simulink library "MotionBaseAdaptersLib"  (R2019b)
settings: Solver=VariableStepAuto  StartTime=0.0  StopTime=10.0  RelTol=1e-3
undefined symbols (not defined in the file): AngularAcceleration, AngularVelocity, ApplyMotion, DiscIntNeverNeededParam, GravitationalAcceleration, LinearAcceleration, LinearVelocity, ManualOrientation, ManualPosition, OrientationDCM, SampleTime, TrackEffectType
libraries: simulink x34, FiltersLib x34, OverridesLib x10, SignalGeneratorsLib x7, LatchesLib x6, TimersLib x5, CoordinateMathOperationsLib x2, MathOperationsLib x2, $bdroot x1
(part 2 of 2)

== system MotionBaseAdaptersLib/MotionBase/MotionBaseAdapter/MotionBaseProcessing/ManualAdjustments/ManualPositionAdjustment1/If Action Subsystem3 ==
  RoughnessProfileFactor : Inport
  Linear Velocity : Inport  Port=2
  RoughnessProfileFrequencyFactor : Inport  Port=3
  Action Port : ActionPort
  AssignZ : Assignment  IndexMode=Zero-based  DiagnosticForDimensions=Warning  IndexOptions=Index vector (dialog)  Indices=2  OutputSizes=1
  Compare To Zero : simulink/Logic and Bit Operations/Compare To Zero  relop=>  OutDataTypeStr=boolean
  Constant : Constant  Value=1/20
  Constant1 : Constant  Value=0.01
  Constant2 : Constant  Value=0
  Data Type Conversion : DataTypeConversion
  Product1 : Product
  Product2 : Product
  Selector : Selector  InputPortWidth=3  IndexOptions=Index vector (dialog)  Indices=1  OutputSizes=1
  Terminator : Terminator
  Triggered Sine Wave Generator : SignalGeneratorsLib/Triggered Sine Wave Generator  SampleTime=SampleTime
      settings: SourceProductName=Signal Generators
  Zeros : Constant  Value=[0 0 0]
  Out1 : Outport  VectorParamsAs1DForOutWhenUnconnected=off
  wires:
  Triggered Sine Wave Generator/1 -> AssignZ/2
  AssignZ/1 -> Out1/1
  Zeros/1 -> AssignZ/1
  Linear Velocity/1 -> Selector/1
  Selector/1 -> Terminator/1
  Compare To Zero/1 -> Data Type Conversion/1
  Data Type Conversion/1 -> Triggered Sine Wave Generator/1
  RoughnessProfileFrequencyFactor/1 -> Product1/2
  Constant/1 -> Product1/1
  Product1/1 -> Triggered Sine Wave Generator/2
  Constant1/1 -> Product2/1
  RoughnessProfileFactor/1 -> Product2/2, Compare To Zero/1
  Product2/1 -> Triggered Sine Wave Generator/3
  Constant2/1 -> Triggered Sine Wave Generator/6, Triggered Sine Wave Generator/5, Triggered Sine Wave Generator/4

== system MotionBaseAdaptersLib/MotionBase/MotionBaseAdapter/MotionBaseProcessing/ManualAdjustments/ManualPositionAdjustment1/If Action Subsystem4 ==
  RoughnessProfileFactor : Inport
  Action Port : ActionPort
  AssignZ : Assignment  IndexMode=Zero-based  DiagnosticForDimensions=Warning  IndexOptions=Index vector (dialog)  Indices=2  OutputSizes=1
  Product : Product
  Scale : Constant  Value=0
  Sine Wave : Sin  Amplitude=0.01  Frequency=20  SampleTime=SampleTime
  Switch : Switch  Criteria=u2 > Threshold
  Zeros : Constant  Value=[0 0 0]
  Out1 : Outport  VectorParamsAs1DForOutWhenUnconnected=off
  wires:
  Product/1 -> AssignZ/2
  Scale/1 -> Switch/3
  Switch/1 -> Product/2
  RoughnessProfileFactor/1 -> Switch/1, Switch/2
  Sine Wave/1 -> Product/1
  AssignZ/1 -> Out1/1
  Zeros/1 -> AssignZ/1

== system MotionBaseAdaptersLib/MotionBase/MotionBaseAdapter/MotionBaseProcessing/ManualAdjustments/ManualPositionAdjustment1/If Action Subsystem5 ==
  Linear Velocity : Inport
  RoughnessProfileFactor : Inport  Port=2
  RoughnessProfileSpeedFactor : Inport  Port=3
  RoughnessProfileSpeedSaturation : Inport  Port=4
  RoughnessProfileFrequencyFactor : Inport  Port=5
  Action Port : ActionPort
  AssignZ : Assignment  IndexMode=Zero-based  DiagnosticForDimensions=Warning  IndexOptions=Index vector (dialog)  Indices=2  OutputSizes=1
  Constant : Constant
  RoughnessGenerator : Subsystem  mask{Variance=0.0001, ClipValue=3, Ts=SampleTime}
      mask prompts: Ts "Simulink:masks:SampleTime_MP"
      mask TypeOptions Ts:
      | Band-Limited
      | White Noise/Ts
      mask DialogControl Ts Prompt: Sample time:
  Selector : Selector  InputPortWidth=3  IndexOptions=Index vector (dialog)  Indices=1  OutputSizes=1
  Zeros : Constant  Value=[0 0 0]
  Out1 : Outport  VectorParamsAs1DForOutWhenUnconnected=off
  wires:
  RoughnessProfileFactor/1 -> RoughnessGenerator/3(RoughnessAmplitudeFactor)
  Zeros/1 -> AssignZ/1
  Selector/1 -> RoughnessGenerator/2(Velocity)  "Forward velocity"
  RoughnessGenerator/1(Out1) -> AssignZ/2
  AssignZ/1 -> Out1/1
  Linear Velocity/1 -> Selector/1
  RoughnessProfileSpeedFactor/1 -> RoughnessGenerator/4(SpeedFactor)
  RoughnessProfileSpeedSaturation/1 -> RoughnessGenerator/5(SpeedSaturation)
  Constant/1 -> RoughnessGenerator/1(Enable)
  RoughnessProfileFrequencyFactor/1 -> RoughnessGenerator/6(RoughnessProfileFrequencyFactor)

== system MotionBaseAdaptersLib/MotionBase/MotionBaseAdapter/MotionBaseProcessing/ManualAdjustments/ManualPositionAdjustment1/If Action Subsystem6 ==
  Linear Velocity : Inport
  RoughnessProfileFactor : Inport  Port=2
  RoughnessProfileSpeedFactor : Inport  Port=3
  RoughnessProfileSpeedSaturation : Inport  Port=4
  RoughnessProfileFrequencyFactor : Inport  Port=5
  Action Port : ActionPort
  AssignZ : Assignment  IndexMode=Zero-based  DiagnosticForDimensions=Warning  IndexOptions=Index vector (dialog)  Indices=2  OutputSizes=1
  Constant : Constant
  RoughnessGenerator : Subsystem  mask{Variance=0.0001, ClipValue=3, Ts=SampleTime}
      mask prompts: Ts "Simulink:masks:SampleTime_MP"
      mask TypeOptions Ts:
      | Band-Limited
      | White Noise/Ts
      mask DialogControl Ts Prompt: Sample time:
  Selector : Selector  InputPortWidth=3  IndexOptions=Index vector (dialog)  Indices=1  OutputSizes=1
  Zeros : Constant  Value=[0 0 0]
  Out1 : Outport  VectorParamsAs1DForOutWhenUnconnected=off
  wires:
  RoughnessProfileSpeedSaturation/1 -> RoughnessGenerator/5(SpeedSaturation)
  RoughnessProfileSpeedFactor/1 -> RoughnessGenerator/4(SpeedFactor)
  Linear Velocity/1 -> Selector/1
  AssignZ/1 -> Out1/1
  RoughnessGenerator/1(Out1) -> AssignZ/2
  Selector/1 -> RoughnessGenerator/2(Velocity)  "Forward velocity"
  Zeros/1 -> AssignZ/1
  RoughnessProfileFactor/1 -> RoughnessGenerator/3(RoughnessAmplitudeFactor)
  Constant/1 -> RoughnessGenerator/1(Enable)
  RoughnessProfileFrequencyFactor/1 -> RoughnessGenerator/6(RoughnessProfileFrequencyFactor)

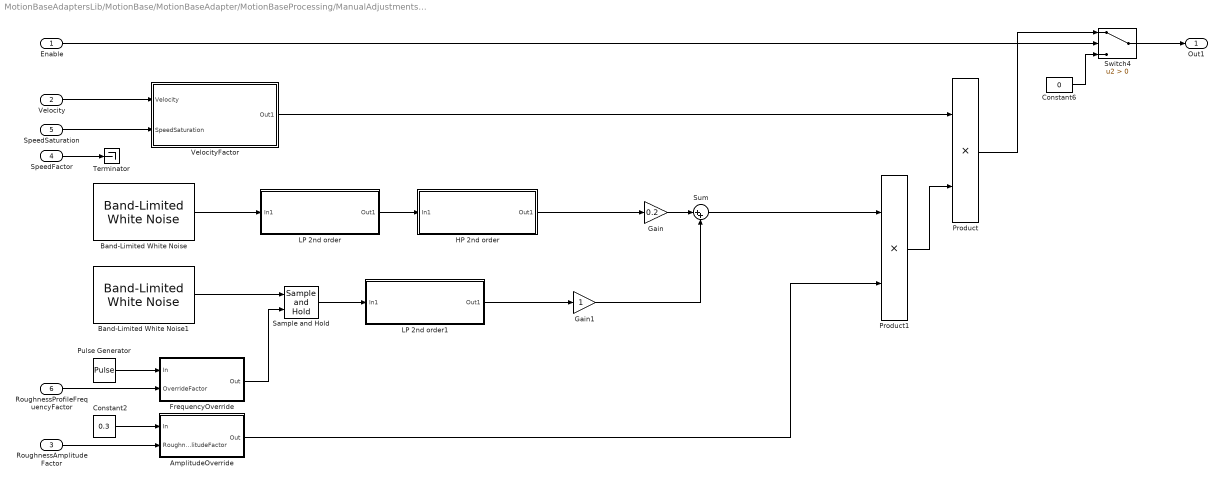
== system MotionBaseAdaptersLib/MotionBase/MotionBaseAdapter/MotionBaseProcessing/ManualAdjustments/ManualPositionAdjustment/DegradedTrackFeel/DegradedRoughnessGenerator ==
  Enable : Inport
  Velocity : Inport  Port=2
  RoughnessAmplitudeFactor : Inport  Port=3
  SpeedFactor : Inport  Port=4
  SpeedSaturation : Inport  Port=5
  RoughnessProfileFrequencyFactor : Inport  Port=6
  AmplitudeOverride : Subsystem
  Band-Limited White Noise : simulink/Sources/Band-Limited White Noise  Cov=[0.1]  Ts=Ts  seed=[23341]
  Band-Limited White Noise1 : simulink/Sources/Band-Limited White Noise  Cov=[0.1]  Ts=SampleTime  seed=[5241]
  Constant2 : Constant  Value=0.3
  Constant6 : Constant  Value=0
  FrequencyOverride : Subsystem
  Gain : Gain  Gain=0.2
  Gain1 : Gain
  HP 2nd order : Subsystem  mask{Frequency=2}
      mask prompts: Frequency "CutOffFrequency"
  LP 2nd order : Subsystem  mask{Frequency=10}
      mask prompts: Frequency "CutOffFrequency"
  LP 2nd order1 : Subsystem  mask{Frequency=5}
      mask prompts: Frequency "CutOffFrequency"
  Product : Product
  Product1 : Product
  Pulse Generator : DiscretePulseGenerator  Period=80  PulseWidth=3  SampleTime=SampleTime
  Sample and Hold : LatchesLib/Sample and Hold  InitialCondition=0  SampleTime=-1
      settings: SourceProductName=Lacthes
  Sum : Sum  Inputs=|++
  Switch4 : Switch  Criteria=u2 > Threshold
  Terminator : Terminator
  VelocityFactor : Subsystem
  Out1 : Outport  VectorParamsAs1DForOutWhenUnconnected=off
  wires:
  VelocityFactor/1(Out1) -> Product/1
  SpeedSaturation/1 -> VelocityFactor/2(SpeedSaturation)
  Velocity/1 -> VelocityFactor/1(Velocity)
  AmplitudeOverride/1(Out) -> Product1/2
  Constant2/1 -> AmplitudeOverride/1(In)
  RoughnessAmplitudeFactor/1 -> AmplitudeOverride/2(RoughnessAmplitudeFactor)
  FrequencyOverride/1(Out) -> Sample and Hold/2
  Pulse Generator/1 -> FrequencyOverride/1(In)
  RoughnessProfileFrequencyFactor/1 -> FrequencyOverride/2(OverrideFactor)
  SpeedFactor/1 -> Terminator/1
  Band-Limited White Noise/1 -> LP 2nd order/1(In1)
  LP 2nd order/1(Out1) -> HP 2nd order/1(In1)
  Product1/1 -> Product/2
  Product/1 -> Switch4/1
  HP 2nd order/1(Out1) -> Gain/1
  Band-Limited White Noise1/1 -> Sample and Hold/1
  LP 2nd order1/1(Out1) -> Gain1/1
  Sum/1 -> Product1/1
  Gain1/1 -> Sum/2
  Gain/1 -> Sum/1
  Sample and Hold/1 -> LP 2nd order1/1(In1)
  Enable/1 -> Switch4/2
  Constant6/1 -> Switch4/3
  Switch4/1 -> Out1/1

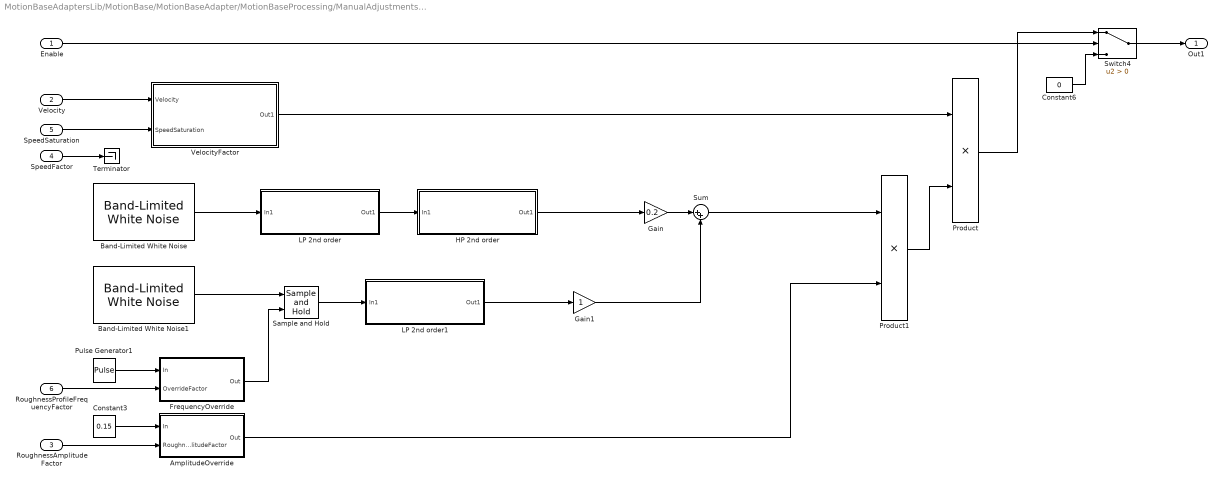
== system MotionBaseAdaptersLib/MotionBase/MotionBaseAdapter/MotionBaseProcessing/ManualAdjustments/ManualPositionAdjustment/StandardTrackFeel/StandardRoughnessGenerator ==
  Enable : Inport
  Velocity : Inport  Port=2
  RoughnessAmplitudeFactor : Inport  Port=3
  SpeedFactor : Inport  Port=4
  SpeedSaturation : Inport  Port=5
  RoughnessProfileFrequencyFactor : Inport  Port=6
  AmplitudeOverride : Subsystem
  Band-Limited White Noise : simulink/Sources/Band-Limited White Noise  Cov=[0.1]  Ts=Ts  seed=[23341]
  Band-Limited White Noise1 : simulink/Sources/Band-Limited White Noise  Cov=[0.1]  Ts=SampleTime  seed=[5241]
  Constant3 : Constant  Value=0.15
  Constant6 : Constant  Value=0
  FrequencyOverride : Subsystem
  Gain : Gain  Gain=0.2
  Gain1 : Gain
  HP 2nd order : Subsystem  mask{Frequency=2}
      mask prompts: Frequency "CutOffFrequency"
  LP 2nd order : Subsystem  mask{Frequency=10}
      mask prompts: Frequency "CutOffFrequency"
  LP 2nd order1 : Subsystem  mask{Frequency=5}
      mask prompts: Frequency "CutOffFrequency"
  Product : Product
  Product1 : Product
  Pulse Generator1 : DiscretePulseGenerator  Period=4800  PulseWidth=80  SampleTime=SampleTime
  Sample and Hold : LatchesLib/Sample and Hold  InitialCondition=0  SampleTime=-1
      settings: SourceProductName=Lacthes
  Sum : Sum  Inputs=|++
  Switch4 : Switch  Criteria=u2 > Threshold
  Terminator : Terminator
  VelocityFactor : Subsystem
  Out1 : Outport  VectorParamsAs1DForOutWhenUnconnected=off
  wires:
  VelocityFactor/1(Out1) -> Product/1
  SpeedSaturation/1 -> VelocityFactor/2(SpeedSaturation)
  Velocity/1 -> VelocityFactor/1(Velocity)
  AmplitudeOverride/1(Out) -> Product1/2
  Constant3/1 -> AmplitudeOverride/1(In)
  RoughnessAmplitudeFactor/1 -> AmplitudeOverride/2(RoughnessAmplitudeFactor)
  FrequencyOverride/1(Out) -> Sample and Hold/2
  Pulse Generator1/1 -> FrequencyOverride/1(In)
  RoughnessProfileFrequencyFactor/1 -> FrequencyOverride/2(OverrideFactor)
  SpeedFactor/1 -> Terminator/1
  Band-Limited White Noise/1 -> LP 2nd order/1(In1)
  LP 2nd order/1(Out1) -> HP 2nd order/1(In1)
  Product1/1 -> Product/2
  Product/1 -> Switch4/1
  HP 2nd order/1(Out1) -> Gain/1
  Band-Limited White Noise1/1 -> Sample and Hold/1
  LP 2nd order1/1(Out1) -> Gain1/1
  Sum/1 -> Product1/1
  Gain1/1 -> Sum/2
  Gain/1 -> Sum/1
  Sample and Hold/1 -> LP 2nd order1/1(In1)
  Enable/1 -> Switch4/2
  Constant6/1 -> Switch4/3
  Switch4/1 -> Out1/1

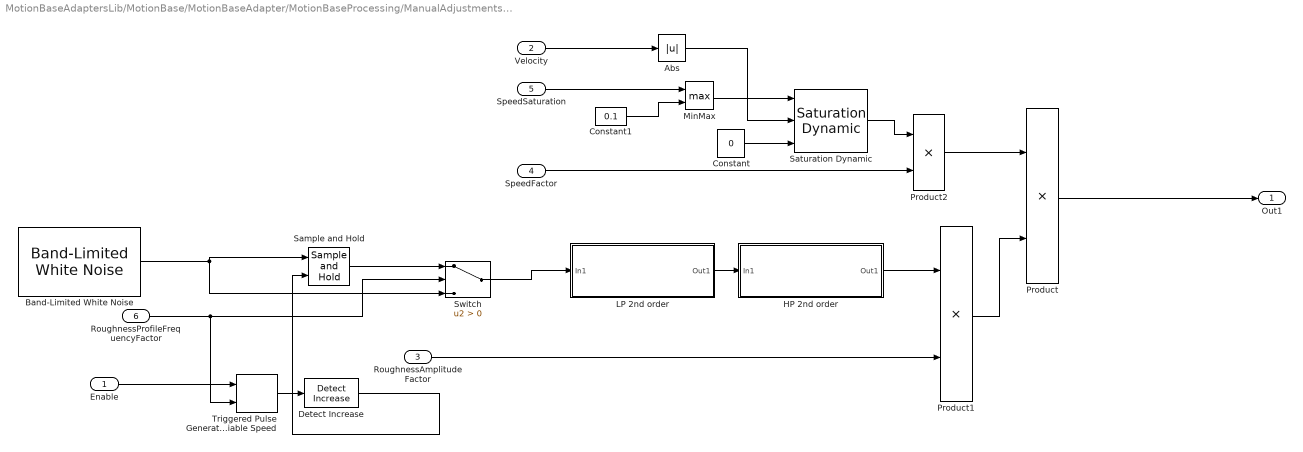
== system MotionBaseAdaptersLib/MotionBase/MotionBaseAdapter/MotionBaseProcessing/ManualAdjustments/ManualPositionAdjustment1/If Action Subsystem/RoughnessGenerator ==
  Enable : Inport
  Velocity : Inport  Port=2
  RoughnessAmplitudeFactor : Inport  Port=3
  SpeedFactor : Inport  Port=4
  SpeedSaturation : Inport  Port=5
  RoughnessProfileFrequencyFactor : Inport  Port=6
  Abs : Abs
  Band-Limited White Noise : simulink/Sources/Band-Limited White Noise  Cov=[0.1]  Ts=Ts  seed=[23341]
  Constant : Constant  Value=0
  Constant1 : Constant  Value=0.1
  Detect Increase : simulink/Logic and Bit Operations/Detect Increase  vinit=0.0  OutDataTypeStr=boolean
  HP 2nd order : Subsystem  mask{Frequency=2}
      mask prompts: Frequency "CutOffFrequency"
  LP 2nd order : Subsystem  mask{Frequency=10}
      mask prompts: Frequency "CutOffFrequency"
  MinMax : MinMax  Function=max  Inputs=2
  Product : Product
  Product1 : Product
  Product2 : Product
  Sample and Hold : LatchesLib/Sample and Hold  InitialCondition=0  SampleTime=-1
      settings: SourceProductName=Lacthes
  Saturation Dynamic : simulink/Discontinuities/Saturation Dynamic  OutMin=[]  OutMax=[]  OutDataTypeStr=Inherit: Same as second input  OutDataType=fixdt(1, 16)  OutScaling=2^-10  DoSatur=off
  Switch : Switch  Criteria=u2 > Threshold
  Triggered Pulse Generator Variable Speed : SignalGeneratorsLib/Triggered Pulse Generator Variable Speed  Amplitude=1  Period=1  PulseWidth=10  PhaseDelay=0  SampleTime=SampleTime
      settings: SourceProductName=Signal Generators
  Out1 : Outport  VectorParamsAs1DForOutWhenUnconnected=off
  wires:
  HP 2nd order/1(Out1) -> Product1/1
  Saturation Dynamic/1 -> Product2/1
  Product/1 -> Out1/1
  Velocity/1 -> Abs/1
  Abs/1 -> Saturation Dynamic/2
  Product1/1 -> Product/2
  LP 2nd order/1(Out1) -> HP 2nd order/1(In1)
  RoughnessAmplitudeFactor/1 -> Product1/2
  SpeedSaturation/1 -> MinMax/1
  Constant/1 -> Saturation Dynamic/3
  Constant1/1 -> MinMax/2
  MinMax/1 -> Saturation Dynamic/1
  SpeedFactor/1 -> Product2/2
  Product2/1 -> Product/1
  Sample and Hold/1 -> Switch/1
  Band-Limited White Noise/1 -> Sample and Hold/1, Switch/3
  Switch/1 -> LP 2nd order/1(In1)
  Detect Increase/1 -> Sample and Hold/2
  Enable/1 -> Triggered Pulse Generator Variable Speed/1
  RoughnessProfileFrequencyFactor/1 -> Triggered Pulse Generator Variable Speed/2, Switch/2
  Triggered Pulse Generator Variable Speed/1 -> Detect Increase/1

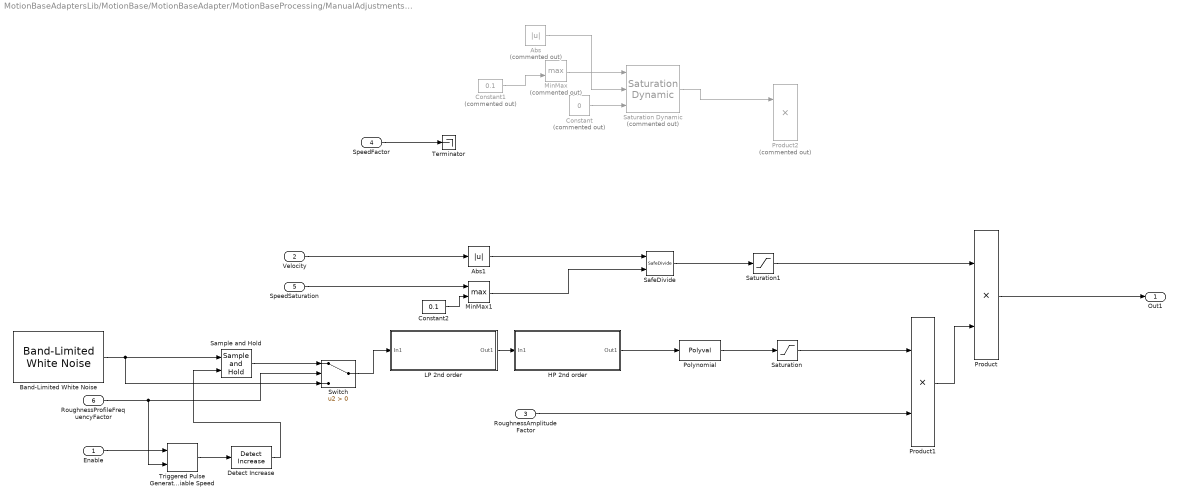
== system MotionBaseAdaptersLib/MotionBase/MotionBaseAdapter/MotionBaseProcessing/ManualAdjustments/ManualPositionAdjustment1/If Action Subsystem1/RoughnessGenerator ==
  Enable : Inport
  Velocity : Inport  Port=2
  RoughnessAmplitudeFactor : Inport  Port=3
  SpeedFactor : Inport  Port=4
  SpeedSaturation : Inport  Port=5
  RoughnessProfileFrequencyFactor : Inport  Port=6
  Abs : Abs  Commented=on
  Abs1 : Abs
  Band-Limited White Noise : simulink/Sources/Band-Limited White Noise  Cov=[0.1]  Ts=Ts  seed=[23341]
  Constant : Constant  Commented=on  Value=0
  Constant1 : Constant  Commented=on  Value=0.1
  Constant2 : Constant  Value=0.1
  Detect Increase : simulink/Logic and Bit Operations/Detect Increase  vinit=0.0  OutDataTypeStr=boolean
  HP 2nd order : Subsystem  mask{Frequency=2}
      mask prompts: Frequency "CutOffFrequency"
  LP 2nd order : Subsystem  mask{Frequency=10}
      mask prompts: Frequency "CutOffFrequency"
  MinMax : MinMax  Commented=on  Function=max  Inputs=2
  MinMax1 : MinMax  Function=max  Inputs=2
  Polynomial : Polyval  Coefs=[1 0 0 0]
  Product : Product
  Product1 : Product
  Product2 : Product  Commented=on
  SafeDivide : MathOperationsLib/SafeDivide
      settings: SourceProductName=Math Operations
  Sample and Hold : LatchesLib/Sample and Hold  InitialCondition=0  SampleTime=-1
      settings: SourceProductName=Lacthes
  Saturation : Saturate  UpperLimit=2.5  LowerLimit=-2.5
  Saturation Dynamic : simulink/Discontinuities/Saturation Dynamic  Commented=on  OutMin=[]  OutMax=[]  OutDataTypeStr=Inherit: Same as second input  OutDataType=fixdt(1, 16)  OutScaling=2^-10  DoSatur=off
  Saturation1 : Saturate  UpperLimit=1  LowerLimit=0
  Switch : Switch  Criteria=u2 > Threshold
  Terminator : Terminator
  Triggered Pulse Generator Variable Speed : SignalGeneratorsLib/Triggered Pulse Generator Variable Speed  Amplitude=1  Period=1  PulseWidth=10  PhaseDelay=0  SampleTime=SampleTime
      settings: SourceProductName=Signal Generators
  Out1 : Outport  VectorParamsAs1DForOutWhenUnconnected=off
  wires:
  Saturation1/1 -> Product/1
  SpeedFactor/1 -> Terminator/1
  MinMax/1 -> Saturation Dynamic/1
  Constant1/1 -> MinMax/2
  Constant/1 -> Saturation Dynamic/3
  RoughnessAmplitudeFactor/1 -> Product1/2
  LP 2nd order/1(Out1) -> HP 2nd order/1(In1)
  Product1/1 -> Product/2
  Abs/1 -> Saturation Dynamic/2
  Product/1 -> Out1/1
  Saturation Dynamic/1 -> Product2/1
  HP 2nd order/1(Out1) -> Polynomial/1
  Polynomial/1 -> Saturation/1
  Saturation/1 -> Product1/1
  Velocity/1 -> Abs1/1
  Abs1/1 -> SafeDivide/1
  SpeedSaturation/1 -> MinMax1/1
  SafeDivide/1 -> Saturation1/1
  MinMax1/1 -> SafeDivide/2
  Constant2/1 -> MinMax1/2
  Sample and Hold/1 -> Switch/1
  Band-Limited White Noise/1 -> Switch/3, Sample and Hold/1
  Switch/1 -> LP 2nd order/1(In1)
  Triggered Pulse Generator Variable Speed/1 -> Detect Increase/1
  Enable/1 -> Triggered Pulse Generator Variable Speed/1
  RoughnessProfileFrequencyFactor/1 -> Triggered Pulse Generator Variable Speed/2, Switch/2
  Detect Increase/1 -> Sample and Hold/2

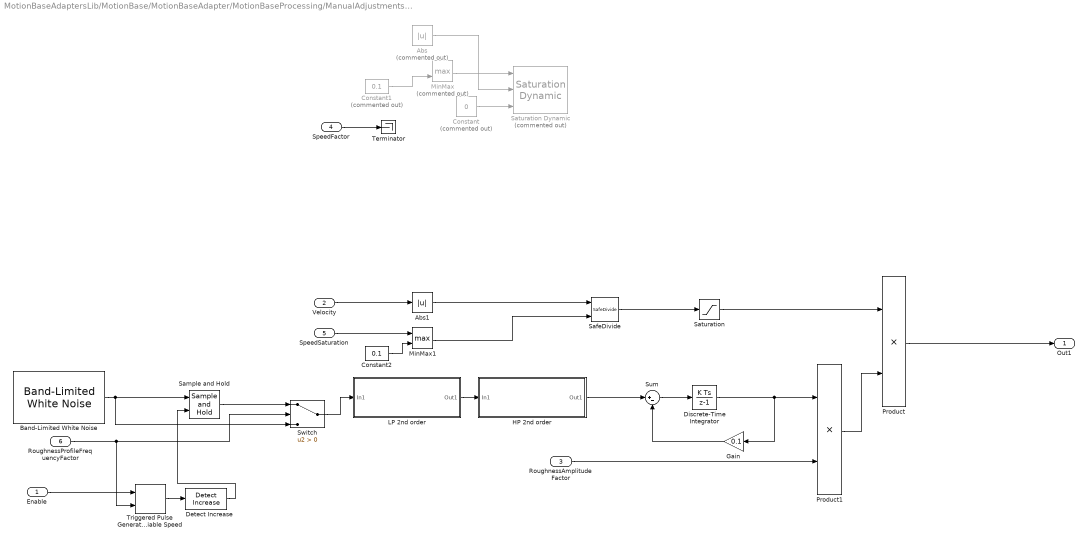
== system MotionBaseAdaptersLib/MotionBase/MotionBaseAdapter/MotionBaseProcessing/ManualAdjustments/ManualPositionAdjustment1/If Action Subsystem5/RoughnessGenerator ==
  Enable : Inport
  Velocity : Inport  Port=2
  RoughnessAmplitudeFactor : Inport  Port=3
  SpeedFactor : Inport  Port=4
  SpeedSaturation : Inport  Port=5
  RoughnessProfileFrequencyFactor : Inport  Port=6
  Abs : Abs  Commented=on
  Abs1 : Abs
  Band-Limited White Noise : simulink/Sources/Band-Limited White Noise  Cov=[0.1]  Ts=Ts  seed=[23341]
  Constant : Constant  Commented=on  Value=0
  Constant1 : Constant  Commented=on  Value=0.1
  Constant2 : Constant  Value=0.1
  Detect Increase : simulink/Logic and Bit Operations/Detect Increase  vinit=0.0  OutDataTypeStr=boolean
  Discrete-Time Integrator : DiscreteIntegrator  SampleTime=-1  ICPrevOutput=DiscIntNeverNeededParam  ICPrevScaledInput=DiscIntNeverNeededParam
  Gain : Gain  Gain=0.1
  HP 2nd order : Subsystem  mask{Frequency=2}
      mask prompts: Frequency "CutOffFrequency"
  LP 2nd order : Subsystem  mask{Frequency=10}
      mask prompts: Frequency "CutOffFrequency"
  MinMax : MinMax  Commented=on  Function=max  Inputs=2
  MinMax1 : MinMax  Function=max  Inputs=2
  Product : Product
  Product1 : Product
  SafeDivide : MathOperationsLib/SafeDivide
      settings: SourceProductName=Math Operations
  Sample and Hold : LatchesLib/Sample and Hold  InitialCondition=0  SampleTime=-1
      settings: SourceProductName=Lacthes
  Saturation : Saturate  UpperLimit=1  LowerLimit=0
  Saturation Dynamic : simulink/Discontinuities/Saturation Dynamic  Commented=on  OutMin=[]  OutMax=[]  OutDataTypeStr=Inherit: Same as second input  OutDataType=fixdt(1, 16)  OutScaling=2^-10  DoSatur=off
  Sum : Sum  Inputs=|+-
  Switch : Switch  Criteria=u2 > Threshold
  Terminator : Terminator
  Triggered Pulse Generator Variable Speed : SignalGeneratorsLib/Triggered Pulse Generator Variable Speed  Amplitude=1  Period=1  PulseWidth=10  PhaseDelay=0  SampleTime=SampleTime
      settings: SourceProductName=Signal Generators
  Out1 : Outport  VectorParamsAs1DForOutWhenUnconnected=off
  wires:
  HP 2nd order/1(Out1) -> Sum/1
  Product/1 -> Out1/1
  Abs/1 -> Saturation Dynamic/2
  Product1/1 -> Product/2
  LP 2nd order/1(Out1) -> HP 2nd order/1(In1)
  Band-Limited White Noise/1 -> Switch/3, Sample and Hold/1
  RoughnessAmplitudeFactor/1 -> Product1/2
  Constant/1 -> Saturation Dynamic/3
  Constant1/1 -> MinMax/2
  MinMax/1 -> Saturation Dynamic/1
  Discrete-Time Integrator/1 -> Gain/1, Product1/1
  Sum/1 -> Discrete-Time Integrator/1
  Gain/1 -> Sum/2
  Velocity/1 -> Abs1/1
  Abs1/1 -> SafeDivide/1
  SpeedSaturation/1 -> MinMax1/1
  Saturation/1 -> Product/1
  SafeDivide/1 -> Saturation/1
  MinMax1/1 -> SafeDivide/2
  Constant2/1 -> MinMax1/2
  SpeedFactor/1 -> Terminator/1
  Detect Increase/1 -> Sample and Hold/2
  Enable/1 -> Triggered Pulse Generator Variable Speed/1
  RoughnessProfileFrequencyFactor/1 -> Triggered Pulse Generator Variable Speed/2, Switch/2
  Sample and Hold/1 -> Switch/1
  Switch/1 -> LP 2nd order/1(In1)
  Triggered Pulse Generator Variable Speed/1 -> Detect Increase/1

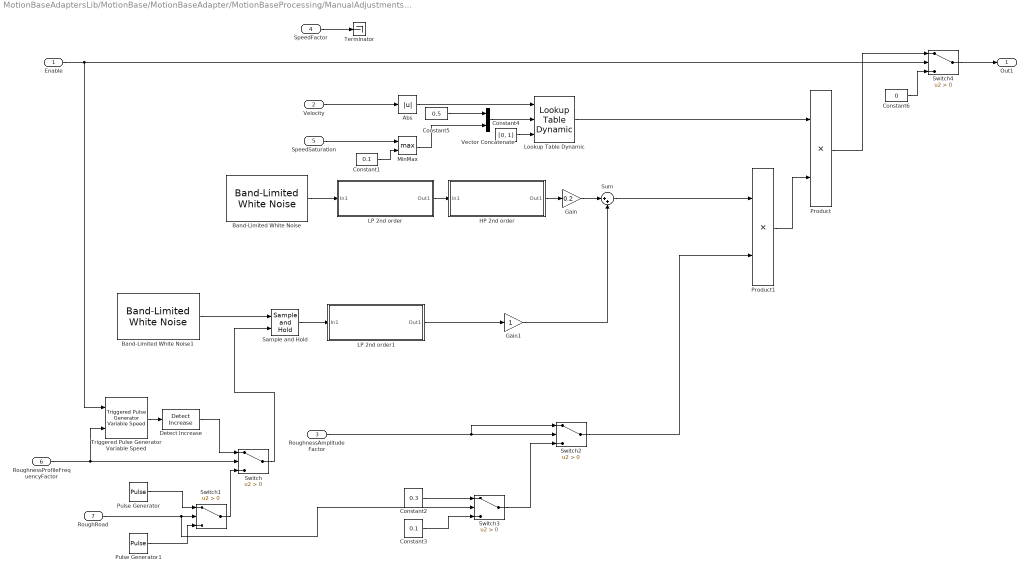
== system MotionBaseAdaptersLib/MotionBase/MotionBaseAdapter/MotionBaseProcessing/ManualAdjustments/ManualPositionAdjustment1/If Action Subsystem6/RoughnessGenerator ==
  Enable : Inport
  Velocity : Inport  Port=2
  RoughnessAmplitudeFactor : Inport  Port=3
  SpeedFactor : Inport  Port=4
  SpeedSaturation : Inport  Port=5
  RoughnessProfileFrequencyFactor : Inport  Port=6
  RoughRoad : Inport  Port=7
  Abs : Abs
  Band-Limited White Noise : simulink/Sources/Band-Limited White Noise  Cov=[0.1]  Ts=Ts  seed=[23341]
  Band-Limited White Noise1 : simulink/Sources/Band-Limited White Noise  Cov=[0.1]  Ts=SampleTime  seed=[5241]
  Constant1 : Constant  Value=0.1
  Constant2 : Constant  Value=0.3
  Constant3 : Constant  Value=0.1
  Constant4 : Constant  Value=[0, 1]
  Constant5 : Constant  Value=0.5
  Constant6 : Constant  Value=0
  Detect Increase : simulink/Logic and Bit Operations/Detect Increase  vinit=0.0  OutDataTypeStr=boolean
  Gain : Gain  Gain=0.2
  Gain1 : Gain
  HP 2nd order : Subsystem  mask{Frequency=2}
      mask prompts: Frequency "CutOffFrequency"
  LP 2nd order : Subsystem  mask{Frequency=10}
      mask prompts: Frequency "CutOffFrequency"
  LP 2nd order1 : Subsystem  mask{Frequency=5}
      mask prompts: Frequency "CutOffFrequency"
  Lookup Table Dynamic : simulink/Lookup Tables/Lookup Table Dynamic  LookUpMeth=Interpolation-Use End Values  OutDataType=fixdt('double')  OutScaling=[]  OutputDataTypeScalingMode=Specify via dialog  OutDataTypeStr=double  DoSatur=off
      settings: SourceProductName=Simulink
  MinMax : MinMax  Function=max  Inputs=2
  Product : Product
  Product1 : Product
  Pulse Generator : DiscretePulseGenerator  Period=80  PulseWidth=3  SampleTime=SampleTime
  Pulse Generator1 : DiscretePulseGenerator  PulseType=Time based  Period=10  SampleTime=SampleTime
  Sample and Hold : LatchesLib/Sample and Hold  InitialCondition=0  SampleTime=-1
      settings: SourceProductName=Lacthes
  Sum : Sum  Inputs=|++
  Switch{,1..4} (5 alike) : Switch  Criteria=u2 > Threshold
  Terminator : Terminator
  Triggered Pulse Generator Variable Speed : SignalGeneratorsLib/Triggered Pulse Generator Variable Speed  Amplitude=1  Period=1  PulseWidth=10  PhaseDelay=0  SampleTime=SampleTime
      settings: SourceProductName=Signal Generators
  Vector Concatenate : Concatenate
  Out1 : Outport  VectorParamsAs1DForOutWhenUnconnected=off
  wires:
  Lookup Table Dynamic/1 -> Product/1
  SpeedFactor/1 -> Terminator/1
  Constant1/1 -> MinMax/2
  SpeedSaturation/1 -> MinMax/1
  RoughnessAmplitudeFactor/1 -> Switch2/1, Switch2/2
  Band-Limited White Noise/1 -> LP 2nd order/1(In1)
  LP 2nd order/1(Out1) -> HP 2nd order/1(In1)
  Product1/1 -> Product/2
  Abs/1 -> Lookup Table Dynamic/1
  Product/1 -> Switch4/1
  HP 2nd order/1(Out1) -> Gain/1
  Band-Limited White Noise1/1 -> Sample and Hold/1
  LP 2nd order1/1(Out1) -> Gain1/1
  Sum/1 -> Product1/1
  Gain1/1 -> Sum/2
  Gain/1 -> Sum/1
  Sample and Hold/1 -> LP 2nd order1/1(In1)
  Triggered Pulse Generator Variable Speed/1 -> Detect Increase/1
  RoughnessProfileFrequencyFactor/1 -> Triggered Pulse Generator Variable Speed/2, Switch/2
  MinMax/1 -> Vector Concatenate/2
  Enable/1 -> Switch4/2, Triggered Pulse Generator Variable Speed/1
  Detect Increase/1 -> Switch/1
  RoughRoad/1 -> Switch3/2, Switch1/2
  Pulse Generator/1 -> Switch1/1
  Pulse Generator1/1 -> Switch1/3
  Switch1/1 -> Switch/3
  Switch/1 -> Sample and Hold/2
  Switch3/1 -> Switch2/3
  Constant2/1 -> Switch3/1
  Constant3/1 -> Switch3/3
  Switch2/1 -> Product1/2
  Velocity/1 -> Abs/1
  Vector Concatenate/1 -> Lookup Table Dynamic/2
  Constant4/1 -> Lookup Table Dynamic/3
  Constant5/1 -> Vector Concatenate/1
  Constant6/1 -> Switch4/3
  Switch4/1 -> Out1/1

== system MotionBaseAdaptersLib/MotionBase/MotionBaseAdapter/MotionBaseProcessing/ManualAdjustments/ManualPositionAdjustment/DegradedTrackFeel/DegradedRoughnessGenerator/AmplitudeOverride ==
  In : Inport
  RoughnessAmplitudeFactor : Inport  Port=2
  Switch2 : Switch  Criteria=u2 > Threshold
  Out : Outport  VectorParamsAs1DForOutWhenUnconnected=off
  wires:
  RoughnessAmplitudeFactor/1 -> Switch2/1, Switch2/2
  In/1 -> Switch2/3
  Switch2/1 -> Out/1

== system MotionBaseAdaptersLib/MotionBase/MotionBaseAdapter/MotionBaseProcessing/ManualAdjustments/ManualPositionAdjustment/DegradedTrackFeel/DegradedRoughnessGenerator/FrequencyOverride ==
  In : Inport
  OverrideFactor : Inport  Port=2
  Compare To Zero : simulink/Logic and Bit Operations/Compare To Zero  relop=>  OutDataTypeStr=boolean
  Detect Increase : simulink/Logic and Bit Operations/Detect Increase  vinit=0.0  OutDataTypeStr=boolean
  Switch : Switch  Criteria=u2 > Threshold
  Triggered Pulse Generator Variable Speed : SignalGeneratorsLib/Triggered Pulse Generator Variable Speed  Amplitude=1  Period=1  PulseWidth=10  PhaseDelay=0  SampleTime=SampleTime
      settings: SourceProductName=Signal Generators
  Out : Outport  VectorParamsAs1DForOutWhenUnconnected=off
  wires:
  Triggered Pulse Generator Variable Speed/1 -> Detect Increase/1
  OverrideFactor/1 -> Compare To Zero/1, Triggered Pulse Generator Variable Speed/2, Switch/2
  Detect Increase/1 -> Switch/1
  In/1 -> Switch/3
  Switch/1 -> Out/1
  Compare To Zero/1 -> Triggered Pulse Generator Variable Speed/1

== system MotionBaseAdaptersLib/MotionBase/MotionBaseAdapter/MotionBaseProcessing/ManualAdjustments/ManualPositionAdjustment/DegradedTrackFeel/DegradedRoughnessGenerator/HP 2nd order ==
  In1 : Inport
  LP Filter : FiltersLib/First Order Low Pass Filter  FilterSpecificationSource=internal  FilterSpecificationType=Specify Cutoff Frequency  FilterSpecificationValue=Frequency  SampleTime=-1
      settings: SourceProductName=SydacTools
  LP Filter1 : FiltersLib/First Order Low Pass Filter  FilterSpecificationSource=internal  FilterSpecificationType=Specify Cutoff Frequency  FilterSpecificationValue=Frequency  SampleTime=-1
      settings: SourceProductName=SydacTools
  Sum : Sum  Inputs=|+-
  Out1 : Outport  VectorParamsAs1DForOutWhenUnconnected=off
  wires:
  LP Filter/1 -> LP Filter1/1
  LP Filter1/1 -> Sum/2
  Sum/1 -> Out1/1
  In1/1 -> Sum/1, LP Filter/1

== system MotionBaseAdaptersLib/MotionBase/MotionBaseAdapter/MotionBaseProcessing/ManualAdjustments/ManualPositionAdjustment/DegradedTrackFeel/DegradedRoughnessGenerator/LP 2nd order ==
  In1 : Inport
  LP Filter : FiltersLib/First Order Low Pass Filter  FilterSpecificationSource=internal  FilterSpecificationType=Specify Cutoff Frequency  FilterSpecificationValue=Frequency  SampleTime=-1
      settings: SourceProductName=SydacTools
  LP Filter1 : FiltersLib/First Order Low Pass Filter  FilterSpecificationSource=internal  FilterSpecificationType=Specify Cutoff Frequency  FilterSpecificationValue=Frequency  SampleTime=-1
      settings: SourceProductName=SydacTools
  Out1 : Outport  VectorParamsAs1DForOutWhenUnconnected=off
  wires:
  LP Filter/1 -> LP Filter1/1
  LP Filter1/1 -> Out1/1
  In1/1 -> LP Filter/1

== system MotionBaseAdaptersLib/MotionBase/MotionBaseAdapter/MotionBaseProcessing/ManualAdjustments/ManualPositionAdjustment/DegradedTrackFeel/DegradedRoughnessGenerator/LP 2nd order1 ==
  In1 : Inport
  LP Filter : FiltersLib/First Order Low Pass Filter  FilterSpecificationSource=internal  FilterSpecificationType=Specify Cutoff Frequency  FilterSpecificationValue=Frequency  SampleTime=-1
      settings: SourceProductName=SydacTools
  LP Filter1 : FiltersLib/First Order Low Pass Filter  FilterSpecificationSource=internal  FilterSpecificationType=Specify Cutoff Frequency  FilterSpecificationValue=Frequency  SampleTime=-1
      settings: SourceProductName=SydacTools
  Out1 : Outport  VectorParamsAs1DForOutWhenUnconnected=off
  wires:
  In1/1 -> LP Filter/1
  LP Filter1/1 -> Out1/1
  LP Filter/1 -> LP Filter1/1

== system MotionBaseAdaptersLib/MotionBase/MotionBaseAdapter/MotionBaseProcessing/ManualAdjustments/ManualPositionAdjustment/DegradedTrackFeel/DegradedRoughnessGenerator/VelocityFactor ==
  Velocity : Inport
  SpeedSaturation : Inport  Port=2
  Abs : Abs
  Constant2 : Constant  Value=0.6
  Constant4 : Constant  Value=[0, 1]
  Constant5 : Constant  Value=0.5
  Lookup Table Dynamic : simulink/Lookup Tables/Lookup Table Dynamic  LookUpMeth=Interpolation-Use End Values  OutDataType=fixdt('double')  OutScaling=[]  OutputDataTypeScalingMode=Specify via dialog  OutDataTypeStr=double  DoSatur=off
      settings: SourceProductName=Simulink
  MinMax : MinMax  Function=max  Inputs=2
  Tuning Factor : OverridesLib/Tuning Factor  DefaultValue=SpeedSaturation  Criteria=u2 > Threshold  Threshold=0
      settings: SourceProductName=Overrides
  Vector Concatenate : Concatenate
  Out1 : Outport  VectorParamsAs1DForOutWhenUnconnected=off
  wires:
  MinMax/1 -> Vector Concatenate/2
  SpeedSaturation/1 -> Tuning Factor/1
  Tuning Factor/1 -> MinMax/1
  Lookup Table Dynamic/1 -> Out1/1
  Constant2/1 -> MinMax/2
  Abs/1 -> Lookup Table Dynamic/1
  Velocity/1 -> Abs/1
  Vector Concatenate/1 -> Lookup Table Dynamic/2
  Constant4/1 -> Lookup Table Dynamic/3
  Constant5/1 -> Vector Concatenate/1

== system MotionBaseAdaptersLib/MotionBase/MotionBaseAdapter/MotionBaseProcessing/ManualAdjustments/ManualPositionAdjustment/StandardTrackFeel/StandardRoughnessGenerator/AmplitudeOverride ==
  In : Inport
  RoughnessAmplitudeFactor : Inport  Port=2
  Switch2 : Switch  Criteria=u2 > Threshold
  Out : Outport  VectorParamsAs1DForOutWhenUnconnected=off
  wires:
  RoughnessAmplitudeFactor/1 -> Switch2/1, Switch2/2
  In/1 -> Switch2/3
  Switch2/1 -> Out/1

== system MotionBaseAdaptersLib/MotionBase/MotionBaseAdapter/MotionBaseProcessing/ManualAdjustments/ManualPositionAdjustment/StandardTrackFeel/StandardRoughnessGenerator/FrequencyOverride ==
  In : Inport
  OverrideFactor : Inport  Port=2
  Compare To Zero : simulink/Logic and Bit Operations/Compare To Zero  relop=>  OutDataTypeStr=boolean
  Detect Increase : simulink/Logic and Bit Operations/Detect Increase  vinit=0.0  OutDataTypeStr=boolean
  Switch : Switch  Criteria=u2 > Threshold
  Triggered Pulse Generator Variable Speed : SignalGeneratorsLib/Triggered Pulse Generator Variable Speed  Amplitude=1  Period=1  PulseWidth=10  PhaseDelay=0  SampleTime=SampleTime
      settings: SourceProductName=Signal Generators
  Out : Outport  VectorParamsAs1DForOutWhenUnconnected=off
  wires:
  Triggered Pulse Generator Variable Speed/1 -> Detect Increase/1
  OverrideFactor/1 -> Compare To Zero/1, Triggered Pulse Generator Variable Speed/2, Switch/2
  Detect Increase/1 -> Switch/1
  In/1 -> Switch/3
  Switch/1 -> Out/1
  Compare To Zero/1 -> Triggered Pulse Generator Variable Speed/1

== system MotionBaseAdaptersLib/MotionBase/MotionBaseAdapter/MotionBaseProcessing/ManualAdjustments/ManualPositionAdjustment/StandardTrackFeel/StandardRoughnessGenerator/HP 2nd order ==
  In1 : Inport
  LP Filter : FiltersLib/First Order Low Pass Filter  FilterSpecificationSource=internal  FilterSpecificationType=Specify Cutoff Frequency  FilterSpecificationValue=Frequency  SampleTime=-1
      settings: SourceProductName=SydacTools
  LP Filter1 : FiltersLib/First Order Low Pass Filter  FilterSpecificationSource=internal  FilterSpecificationType=Specify Cutoff Frequency  FilterSpecificationValue=Frequency  SampleTime=-1
      settings: SourceProductName=SydacTools
  Sum : Sum  Inputs=|+-
  Out1 : Outport  VectorParamsAs1DForOutWhenUnconnected=off
  wires:
  LP Filter/1 -> LP Filter1/1
  LP Filter1/1 -> Sum/2
  Sum/1 -> Out1/1
  In1/1 -> Sum/1, LP Filter/1

== system MotionBaseAdaptersLib/MotionBase/MotionBaseAdapter/MotionBaseProcessing/ManualAdjustments/ManualPositionAdjustment/StandardTrackFeel/StandardRoughnessGenerator/LP 2nd order ==
  In1 : Inport
  LP Filter : FiltersLib/First Order Low Pass Filter  FilterSpecificationSource=internal  FilterSpecificationType=Specify Cutoff Frequency  FilterSpecificationValue=Frequency  SampleTime=-1
      settings: SourceProductName=SydacTools
  LP Filter1 : FiltersLib/First Order Low Pass Filter  FilterSpecificationSource=internal  FilterSpecificationType=Specify Cutoff Frequency  FilterSpecificationValue=Frequency  SampleTime=-1
      settings: SourceProductName=SydacTools
  Out1 : Outport  VectorParamsAs1DForOutWhenUnconnected=off
  wires:
  LP Filter/1 -> LP Filter1/1
  LP Filter1/1 -> Out1/1
  In1/1 -> LP Filter/1

== system MotionBaseAdaptersLib/MotionBase/MotionBaseAdapter/MotionBaseProcessing/ManualAdjustments/ManualPositionAdjustment/StandardTrackFeel/StandardRoughnessGenerator/LP 2nd order1 ==
  In1 : Inport
  LP Filter : FiltersLib/First Order Low Pass Filter  FilterSpecificationSource=internal  FilterSpecificationType=Specify Cutoff Frequency  FilterSpecificationValue=Frequency  SampleTime=-1
      settings: SourceProductName=SydacTools
  LP Filter1 : FiltersLib/First Order Low Pass Filter  FilterSpecificationSource=internal  FilterSpecificationType=Specify Cutoff Frequency  FilterSpecificationValue=Frequency  SampleTime=-1
      settings: SourceProductName=SydacTools
  Out1 : Outport  VectorParamsAs1DForOutWhenUnconnected=off
  wires:
  In1/1 -> LP Filter/1
  LP Filter1/1 -> Out1/1
  LP Filter/1 -> LP Filter1/1

== system MotionBaseAdaptersLib/MotionBase/MotionBaseAdapter/MotionBaseProcessing/ManualAdjustments/ManualPositionAdjustment/StandardTrackFeel/StandardRoughnessGenerator/VelocityFactor ==
  Velocity : Inport
  SpeedSaturation : Inport  Port=2
  Abs : Abs
  Constant1 : Constant  Value=0.6
  Constant4 : Constant  Value=[0, 1]
  Constant5 : Constant  Value=0.5
  Lookup Table Dynamic : simulink/Lookup Tables/Lookup Table Dynamic  LookUpMeth=Interpolation-Use End Values  OutDataType=fixdt('double')  OutScaling=[]  OutputDataTypeScalingMode=Specify via dialog  OutDataTypeStr=double  DoSatur=off
      settings: SourceProductName=Simulink
  MinMax : MinMax  Function=max  Inputs=2
  Tuning Factor : OverridesLib/Tuning Factor  DefaultValue=SpeedSaturation  Criteria=u2 > Threshold  Threshold=0
      settings: SourceProductName=Overrides
  Vector Concatenate : Concatenate
  Out1 : Outport  VectorParamsAs1DForOutWhenUnconnected=off
  wires:
  SpeedSaturation/1 -> Tuning Factor/1
  Lookup Table Dynamic/1 -> Out1/1
  Constant1/1 -> MinMax/2
  Tuning Factor/1 -> MinMax/1
  Abs/1 -> Lookup Table Dynamic/1
  MinMax/1 -> Vector Concatenate/2
  Velocity/1 -> Abs/1
  Vector Concatenate/1 -> Lookup Table Dynamic/2
  Constant4/1 -> Lookup Table Dynamic/3
  Constant5/1 -> Vector Concatenate/1

== system MotionBaseAdaptersLib/MotionBase/MotionBaseAdapter/MotionBaseProcessing/ManualAdjustments/ManualPositionAdjustment1/If Action Subsystem/RoughnessGenerator/HP 2nd order ==
  In1 : Inport
  LP Filter : FiltersLib/First Order Low Pass Filter  FilterSpecificationSource=internal  FilterSpecificationType=Specify Cutoff Frequency  FilterSpecificationValue=Frequency  SampleTime=-1
      settings: SourceProductName=SydacTools
  LP Filter1 : FiltersLib/First Order Low Pass Filter  FilterSpecificationSource=internal  FilterSpecificationType=Specify Cutoff Frequency  FilterSpecificationValue=Frequency  SampleTime=-1
      settings: SourceProductName=SydacTools
  Sum : Sum  Inputs=|+-
  Out1 : Outport  VectorParamsAs1DForOutWhenUnconnected=off
  wires:
  In1/1 -> LP Filter/1, Sum/1
  Sum/1 -> Out1/1
  LP Filter1/1 -> Sum/2
  LP Filter/1 -> LP Filter1/1

== system MotionBaseAdaptersLib/MotionBase/MotionBaseAdapter/MotionBaseProcessing/ManualAdjustments/ManualPositionAdjustment1/If Action Subsystem/RoughnessGenerator/LP 2nd order ==
  In1 : Inport
  LP Filter : FiltersLib/First Order Low Pass Filter  FilterSpecificationSource=internal  FilterSpecificationType=Specify Cutoff Frequency  FilterSpecificationValue=Frequency  SampleTime=-1
      settings: SourceProductName=SydacTools
  LP Filter1 : FiltersLib/First Order Low Pass Filter  FilterSpecificationSource=internal  FilterSpecificationType=Specify Cutoff Frequency  FilterSpecificationValue=Frequency  SampleTime=-1
      settings: SourceProductName=SydacTools
  Out1 : Outport  VectorParamsAs1DForOutWhenUnconnected=off
  wires:
  In1/1 -> LP Filter/1
  LP Filter1/1 -> Out1/1
  LP Filter/1 -> LP Filter1/1

== system MotionBaseAdaptersLib/MotionBase/MotionBaseAdapter/MotionBaseProcessing/ManualAdjustments/ManualPositionAdjustment1/If Action Subsystem1/RoughnessGenerator/HP 2nd order ==
  In1 : Inport
  LP Filter : FiltersLib/First Order Low Pass Filter  FilterSpecificationSource=internal  FilterSpecificationType=Specify Cutoff Frequency  FilterSpecificationValue=Frequency  SampleTime=-1
      settings: SourceProductName=SydacTools
  LP Filter1 : FiltersLib/First Order Low Pass Filter  FilterSpecificationSource=internal  FilterSpecificationType=Specify Cutoff Frequency  FilterSpecificationValue=Frequency  SampleTime=-1
      settings: SourceProductName=SydacTools
  Sum : Sum  Inputs=|+-
  Out1 : Outport  VectorParamsAs1DForOutWhenUnconnected=off
  wires:
  LP Filter/1 -> LP Filter1/1
  LP Filter1/1 -> Sum/2
  Sum/1 -> Out1/1
  In1/1 -> Sum/1, LP Filter/1

== system MotionBaseAdaptersLib/MotionBase/MotionBaseAdapter/MotionBaseProcessing/ManualAdjustments/ManualPositionAdjustment1/If Action Subsystem1/RoughnessGenerator/LP 2nd order ==
  In1 : Inport
  LP Filter : FiltersLib/First Order Low Pass Filter  FilterSpecificationSource=internal  FilterSpecificationType=Specify Cutoff Frequency  FilterSpecificationValue=Frequency  SampleTime=-1
      settings: SourceProductName=SydacTools
  LP Filter1 : FiltersLib/First Order Low Pass Filter  FilterSpecificationSource=internal  FilterSpecificationType=Specify Cutoff Frequency  FilterSpecificationValue=Frequency  SampleTime=-1
      settings: SourceProductName=SydacTools
  Out1 : Outport  VectorParamsAs1DForOutWhenUnconnected=off
  wires:
  LP Filter/1 -> LP Filter1/1
  LP Filter1/1 -> Out1/1
  In1/1 -> LP Filter/1

== system MotionBaseAdaptersLib/MotionBase/MotionBaseAdapter/MotionBaseProcessing/ManualAdjustments/ManualPositionAdjustment1/If Action Subsystem5/RoughnessGenerator/HP 2nd order ==
  In1 : Inport
  LP Filter : FiltersLib/First Order Low Pass Filter  FilterSpecificationSource=internal  FilterSpecificationType=Specify Cutoff Frequency  FilterSpecificationValue=Frequency  SampleTime=-1
      settings: SourceProductName=SydacTools
  LP Filter1 : FiltersLib/First Order Low Pass Filter  FilterSpecificationSource=internal  FilterSpecificationType=Specify Cutoff Frequency  FilterSpecificationValue=Frequency  SampleTime=-1
      settings: SourceProductName=SydacTools
  Sum : Sum  Inputs=|+-
  Out1 : Outport  VectorParamsAs1DForOutWhenUnconnected=off
  wires:
  In1/1 -> LP Filter/1, Sum/1
  Sum/1 -> Out1/1
  LP Filter1/1 -> Sum/2
  LP Filter/1 -> LP Filter1/1

== system MotionBaseAdaptersLib/MotionBase/MotionBaseAdapter/MotionBaseProcessing/ManualAdjustments/ManualPositionAdjustment1/If Action Subsystem5/RoughnessGenerator/LP 2nd order ==
  In1 : Inport
  LP Filter : FiltersLib/First Order Low Pass Filter  FilterSpecificationSource=internal  FilterSpecificationType=Specify Cutoff Frequency  FilterSpecificationValue=Frequency  SampleTime=-1
      settings: SourceProductName=SydacTools
  LP Filter1 : FiltersLib/First Order Low Pass Filter  FilterSpecificationSource=internal  FilterSpecificationType=Specify Cutoff Frequency  FilterSpecificationValue=Frequency  SampleTime=-1
      settings: SourceProductName=SydacTools
  Out1 : Outport  VectorParamsAs1DForOutWhenUnconnected=off
  wires:
  In1/1 -> LP Filter/1
  LP Filter1/1 -> Out1/1
  LP Filter/1 -> LP Filter1/1

== system MotionBaseAdaptersLib/MotionBase/MotionBaseAdapter/MotionBaseProcessing/ManualAdjustments/ManualPositionAdjustment1/If Action Subsystem6/RoughnessGenerator/HP 2nd order ==
  In1 : Inport
  LP Filter : FiltersLib/First Order Low Pass Filter  FilterSpecificationSource=internal  FilterSpecificationType=Specify Cutoff Frequency  FilterSpecificationValue=Frequency  SampleTime=-1
      settings: SourceProductName=SydacTools
  LP Filter1 : FiltersLib/First Order Low Pass Filter  FilterSpecificationSource=internal  FilterSpecificationType=Specify Cutoff Frequency  FilterSpecificationValue=Frequency  SampleTime=-1
      settings: SourceProductName=SydacTools
  Sum : Sum  Inputs=|+-
  Out1 : Outport  VectorParamsAs1DForOutWhenUnconnected=off
  wires:
  LP Filter/1 -> LP Filter1/1
  LP Filter1/1 -> Sum/2
  Sum/1 -> Out1/1
  In1/1 -> Sum/1, LP Filter/1

== system MotionBaseAdaptersLib/MotionBase/MotionBaseAdapter/MotionBaseProcessing/ManualAdjustments/ManualPositionAdjustment1/If Action Subsystem6/RoughnessGenerator/LP 2nd order ==
  In1 : Inport
  LP Filter : FiltersLib/First Order Low Pass Filter  FilterSpecificationSource=internal  FilterSpecificationType=Specify Cutoff Frequency  FilterSpecificationValue=Frequency  SampleTime=-1
      settings: SourceProductName=SydacTools
  LP Filter1 : FiltersLib/First Order Low Pass Filter  FilterSpecificationSource=internal  FilterSpecificationType=Specify Cutoff Frequency  FilterSpecificationValue=Frequency  SampleTime=-1
      settings: SourceProductName=SydacTools
  Out1 : Outport  VectorParamsAs1DForOutWhenUnconnected=off
  wires:
  LP Filter/1 -> LP Filter1/1
  LP Filter1/1 -> Out1/1
  In1/1 -> LP Filter/1

== system MotionBaseAdaptersLib/MotionBase/MotionBaseAdapter/MotionBaseProcessing/ManualAdjustments/ManualPositionAdjustment1/If Action Subsystem6/RoughnessGenerator/LP 2nd order1 ==
  In1 : Inport
  LP Filter : FiltersLib/First Order Low Pass Filter  FilterSpecificationSource=internal  FilterSpecificationType=Specify Cutoff Frequency  FilterSpecificationValue=Frequency  SampleTime=-1
      settings: SourceProductName=SydacTools
  LP Filter1 : FiltersLib/First Order Low Pass Filter  FilterSpecificationSource=internal  FilterSpecificationType=Specify Cutoff Frequency  FilterSpecificationValue=Frequency  SampleTime=-1
      settings: SourceProductName=SydacTools
  Out1 : Outport  VectorParamsAs1DForOutWhenUnconnected=off
  wires:
  In1/1 -> LP Filter/1
  LP Filter1/1 -> Out1/1
  LP Filter/1 -> LP Filter1/1
